simulink model "fit6DoF_th"  (R2018b)
settings: Solver=VariableStepAuto  StartTime=0.0  StopTime=0  RelTol=1e-3
values from neighbouring files (symbols this model uses):
  D = DBdyTrue    [fit6DoFDoF_ts1.m]    (also in perfIndx.m = rotMat * D; perfIndx_ts.m = [d1(:) d2(:) d3(:) d4(:)]; perfIndx_ts1.m = [d1(:) d2(:) d3(:) d4(:)])
  R = [r1(:) r2(:) r3(:) r4(:)]    [perfIndx_ts.m]    (also in perfIndx_ts1.m)
  U = [u1(:) u2(:) u3(:) u4(:)]    [perfIndx_ts.m]    (also in perfIndx_ts1.m)
  w = ones([1 numDots])    [fit6DoFDoF_ts1.m]    (also in perfIndx_ts.m = [1 1 1 1]; perfIndx_ts1.m = [1 1 1 1]; perfIndx_ts2.m)
libraries: fit6DoF x1
settings Model: Creator=M.Cobb  LastModifiedBy=M.Cobb

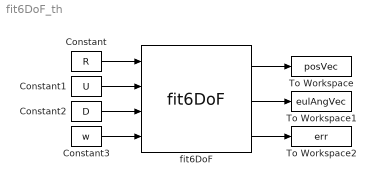
== system fit6DoF_th ==
  Constant : Constant  Value=R
  Constant1 : Constant  Value=U
  Constant2 : Constant  Value=D
  Constant3 : Constant  Value=w
  To Workspace : ToWorkspace  VariableName=posVec  SaveFormat=Timeseries  SampleTime=-1
  To Workspace1 : ToWorkspace  VariableName=eulAngVec  SaveFormat=Timeseries  SampleTime=-1
  To Workspace2 : ToWorkspace  VariableName=err  SaveFormat=Timeseries  SampleTime=-1
  fit6DoF : fit6DoF/fit6DoF  initPosVec=[0 0 50]  initEulAng=[0 0 0]*pi/180  HInvInit=eye(6)  maxIBFGS=1000  posTolBFGS=0.05  angTolBFGS=0.05*pi/180  dxPos=0.0001*[1 1 1]  dxEul=0.01*[1 1 1]*pi/180  stepSize=1e-4  maxIBP=1000  maxIGS=1000  posTolGS=0.05  angTolGS=0.05*pi/180
  wires:
  Constant/1 -> fit6DoF/1
  Constant1/1 -> fit6DoF/2
  Constant2/1 -> fit6DoF/3
  Constant3/1 -> fit6DoF/4
  fit6DoF/1 -> To Workspace/1
  fit6DoF/2 -> To Workspace1/1
  fit6DoF/3 -> To Workspace2/1
